simulink model "prueba"  (R2023a)
settings: Solver=VariableStepAuto  StartTime=0.0  StopTime=1.6  RelTol=1e-3
values from neighbouring files (symbols this model uses):
  Fg = 0.6263    [datos_planta.m]
  Jb = (305490.04e-12)*0.1    (= 3.0549004e-08)    [datos_planta.m]
  m = 0.06385    [datos_planta.m]
  Rr = 21    [datos_planta.m]
settings Model: Creator=hiago.sodre  LastModifiedBy=hiago.sodre

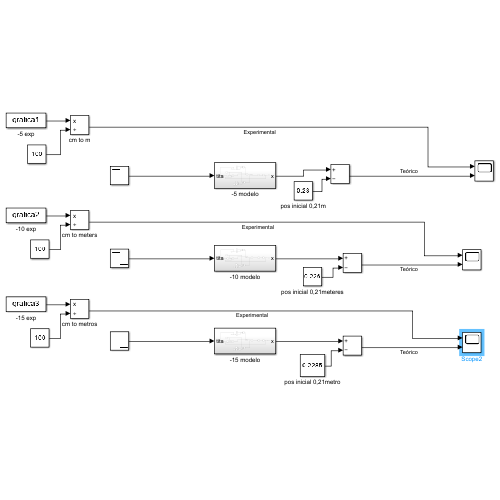
[thumbnail: Simulink's stored preview of the top-level diagram]
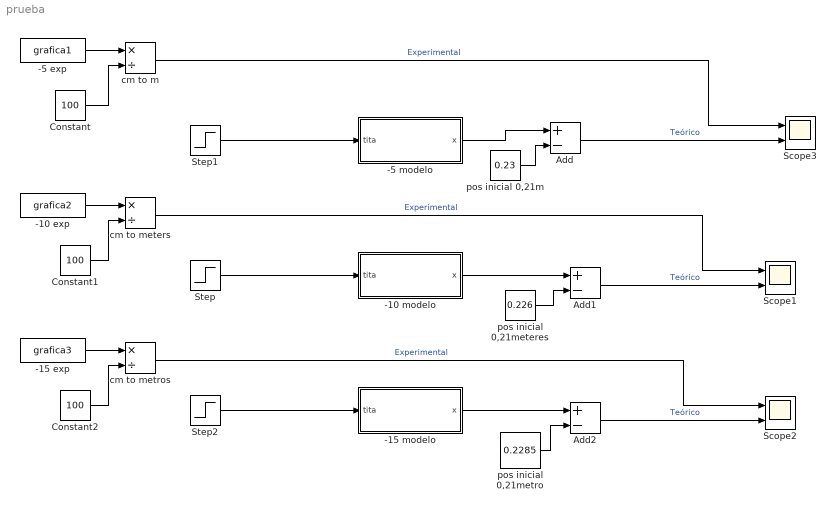
== system prueba ==
  -10 exp : FromWorkspace  VariableName=grafica2
  -10 modelo : Subsystem
  -15 exp : FromWorkspace  VariableName=grafica3
  -15 modelo : Subsystem
  -5 exp : FromWorkspace  VariableName=grafica1
  -5 modelo : Subsystem
  Add : Sum  Inputs=+-
  Add1 : Sum  Inputs=+-
  Add2 : Sum  Inputs=+-
  Constant : Constant  Value=100
  Constant1 : Constant  Value=100
  Constant2 : Constant  Value=100
  Scope1 : Scope  NumInputPorts=2
  Scope2 : Scope  NumInputPorts=2
  Scope3 : Scope  NumInputPorts=2
  Step : Step  Time=0.568  After=-0.1745  SampleTime=0
  Step1 : Step  Time=0.617  After=-0.14  SampleTime=0
  Step2 : Step  Time=0.817  After=-0.2618  SampleTime=0
  cm to m : Product  Inputs=*/
  cm to meters : Product  Inputs=*/
  cm to metros : Product  Inputs=*/
  pos inicial 0,21m : Constant  Value=0.23
  pos inicial 0,21meteres : Constant  Value=0.226
  pos inicial 0,21metro : Constant  Value=0.2285
  wires:
  -5 modelo/1(x) -> Add/1
  Step2/1 -> -15 modelo/1(tita)
  Step/1 -> -10 modelo/1(tita)
  Step1/1 -> -5 modelo/1(tita)
  -5 exp/1 -> cm to m/1
  Constant/1 -> cm to m/2
  pos inicial 0,21m/1 -> Add/2
  pos inicial 0,21meteres/1 -> Add1/2
  -10 modelo/1(x) -> Add1/1
  -15 modelo/1(x) -> Add2/1
  pos inicial 0,21metro/1 -> Add2/2
  Constant1/1 -> cm to meters/2
  -10 exp/1 -> cm to meters/1
  Constant2/1 -> cm to metros/2
  cm to m/1 -> Scope3/1  "Experimental"
  Add/1 -> Scope3/2  "Teórico"
  cm to meters/1 -> Scope1/1  "Experimental"
  Add1/1 -> Scope1/2  "Teórico"
  -15 exp/1 -> cm to metros/1
  cm to metros/1 -> Scope2/1  "Experimental"
  Add2/1 -> Scope2/2  "Teórico"

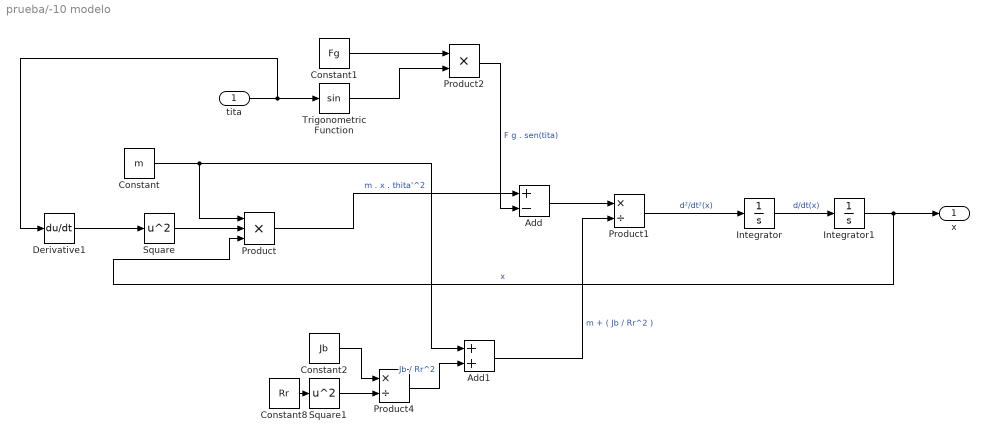
== system prueba/-10 modelo ==
  tita : Inport
  Add : Sum  Inputs=+-
  Add1 : Sum
  Constant : Constant  Value=m
  Constant1 : Constant  Value=Fg
  Constant2 : Constant  Value=Jb
  Constant8 : Constant  Value=Rr
  Derivative1 : Derivative
  Integrator : Integrator
  Integrator1 : Integrator
  Product : Product  Inputs=3
  Product1 : Product  Inputs=*/
  Product2 : Product
  Product4 : Product  Inputs=*/
  Square : Math  Operator=square
  Square1 : Math  Operator=square
  Trigonometric Function : Trigonometry
  x : Outport
  wires:
  Add/1 -> Product1/1
  Square/1 -> Product/2
  Integrator/1 -> Integrator1/1  "d/dt(x)"
  Integrator1/1 -> x/1, Product/3  "x"
  Product/1 -> Add/1  "m . x . thita'^2"
  Constant1/1 -> Product2/1
  Product2/1 -> Add/2  "F g . sen(tita)"
  Product1/1 -> Integrator/1  "d²/dt²(x)"
  Product4/1 -> Add1/2  "Jb / Rr^2"
  Constant2/1 -> Product4/1
  Constant/1 -> Add1/1, Product/1
  Square1/1 -> Product4/2
  Constant8/1 -> Square1/1
  Add1/1 -> Product1/2  "m + ( Jb / Rr^2 )"
  Trigonometric Function/1 -> Product2/2
  tita/1 -> Derivative1/1, Trigonometric Function/1
  Derivative1/1 -> Square/1

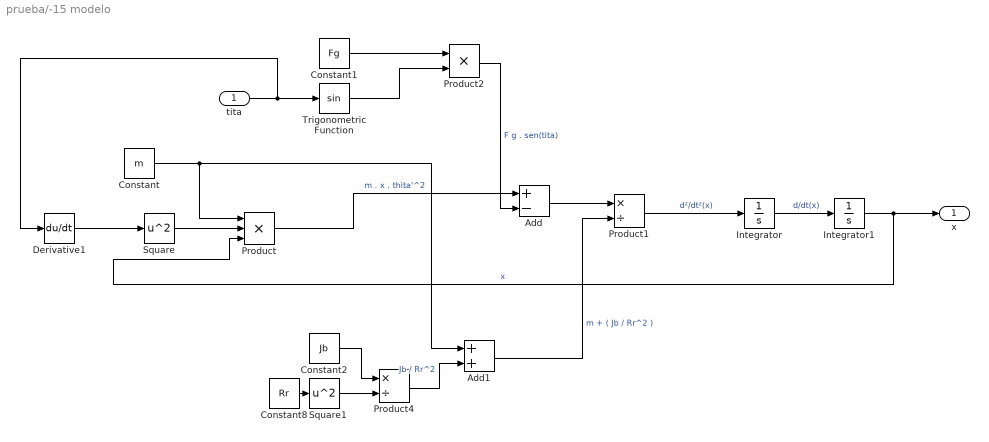
== system prueba/-15 modelo ==
  tita : Inport
  Add : Sum  Inputs=+-
  Add1 : Sum
  Constant : Constant  Value=m
  Constant1 : Constant  Value=Fg
  Constant2 : Constant  Value=Jb
  Constant8 : Constant  Value=Rr
  Derivative1 : Derivative
  Integrator : Integrator
  Integrator1 : Integrator
  Product : Product  Inputs=3
  Product1 : Product  Inputs=*/
  Product2 : Product
  Product4 : Product  Inputs=*/
  Square : Math  Operator=square
  Square1 : Math  Operator=square
  Trigonometric Function : Trigonometry
  x : Outport
  wires:
  Add/1 -> Product1/1
  Square/1 -> Product/2
  Integrator/1 -> Integrator1/1  "d/dt(x)"
  Integrator1/1 -> x/1, Product/3  "x"
  Product/1 -> Add/1  "m . x . thita'^2"
  Constant1/1 -> Product2/1
  Product2/1 -> Add/2  "F g . sen(tita)"
  Product1/1 -> Integrator/1  "d²/dt²(x)"
  Product4/1 -> Add1/2  "Jb / Rr^2"
  Constant2/1 -> Product4/1
  Constant/1 -> Add1/1, Product/1
  Square1/1 -> Product4/2
  Constant8/1 -> Square1/1
  Add1/1 -> Product1/2  "m + ( Jb / Rr^2 )"
  Trigonometric Function/1 -> Product2/2
  tita/1 -> Derivative1/1, Trigonometric Function/1
  Derivative1/1 -> Square/1

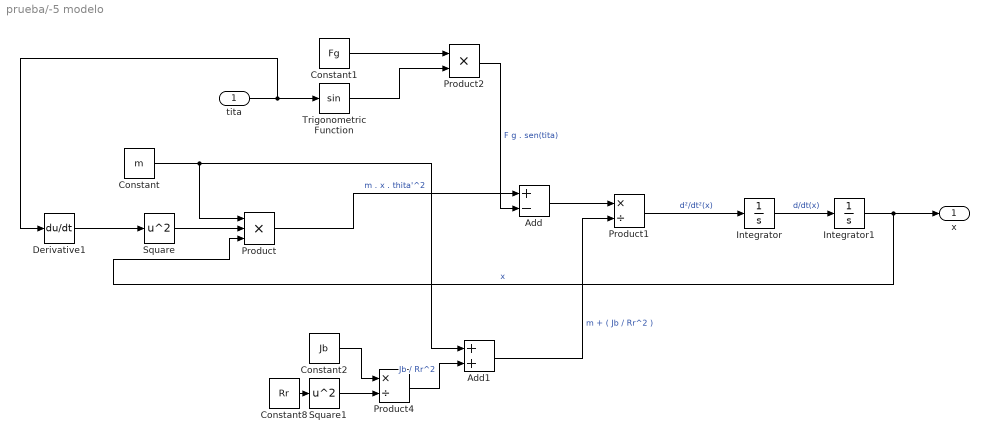
== system prueba/-5 modelo ==
  tita : Inport
  Add : Sum  Inputs=+-
  Add1 : Sum
  Constant : Constant  Value=m
  Constant1 : Constant  Value=Fg
  Constant2 : Constant  Value=Jb
  Constant8 : Constant  Value=Rr
  Derivative1 : Derivative
  Integrator : Integrator
  Integrator1 : Integrator
  Product : Product  Inputs=3
  Product1 : Product  Inputs=*/
  Product2 : Product
  Product4 : Product  Inputs=*/
  Square : Math  Operator=square
  Square1 : Math  Operator=square
  Trigonometric Function : Trigonometry
  x : Outport
  wires:
  Add/1 -> Product1/1
  Square/1 -> Product/2
  Integrator/1 -> Integrator1/1  "d/dt(x)"
  Integrator1/1 -> x/1, Product/3  "x"
  Product/1 -> Add/1  "m . x . thita'^2"
  Constant1/1 -> Product2/1
  Product2/1 -> Add/2  "F g . sen(tita)"
  Product1/1 -> Integrator/1  "d²/dt²(x)"
  Product4/1 -> Add1/2  "Jb / Rr^2"
  Constant2/1 -> Product4/1
  Constant/1 -> Add1/1, Product/1
  Square1/1 -> Product4/2
  Constant8/1 -> Square1/1
  Add1/1 -> Product1/2  "m + ( Jb / Rr^2 )"
  Trigonometric Function/1 -> Product2/2
  tita/1 -> Derivative1/1, Trigonometric Function/1
  Derivative1/1 -> Square/1
